simulink library "INT_StSys_Strt"  (R2016b)
settings: Solver=VariableStepAuto  StartTime=0.0  StopTime=10.0  RelTol=1e-3
settings Model: Creator=Administrator  LastModifiedBy=Administrator

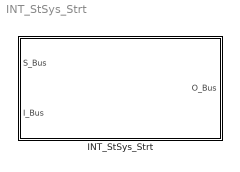
== system INT_StSys_Strt ==
  INT_StSys_Strt : Subsystem

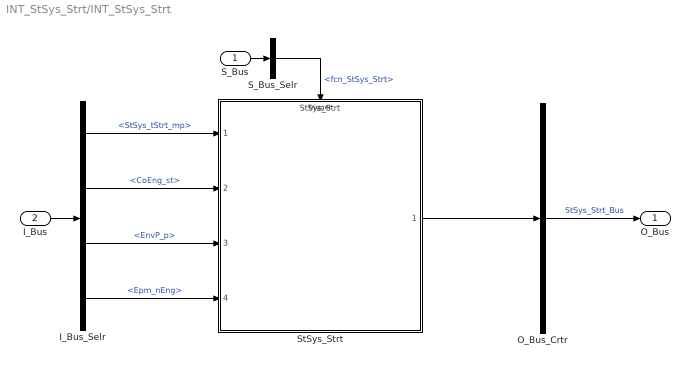
== system INT_StSys_Strt/INT_StSys_Strt ==
  S_Bus : Inport
  I_Bus : Inport  Port=2
  I_Bus_Selr : BusSelector  OutputSignals=StSys_tStrt_mp,CoEng_st,EnvP_p,Epm_nEng
  O_Bus_Crtr : BusCreator  Inputs=1
  S_Bus_Selr : BusSelector  OutputSignals=fcn_StSys_Strt
  StSys_Strt : ModelReference  ModelNameDialog=StSys_Strt  SimulationMode=Normal  ModelReferenceVersion=1.20  TriggerPortName=function  TriggerPortTriggerType=function-call  TriggerPortStatesWhenEnabling=held
  O_Bus : Outport
  wires:
  S_Bus_Selr/1 -> StSys_Strt/Trigger  "<fcn_StSys_Strt>"
  S_Bus/1 -> S_Bus_Selr/1
  I_Bus/1 -> I_Bus_Selr/1
  I_Bus_Selr/1 -> StSys_Strt/1  "<StSys_tStrt_mp>"
  I_Bus_Selr/2 -> StSys_Strt/2  "<CoEng_st>"
  I_Bus_Selr/3 -> StSys_Strt/3  "<EnvP_p>"
  I_Bus_Selr/4 -> StSys_Strt/4  "<Epm_nEng>"
  O_Bus_Crtr/1 -> O_Bus/1  "StSys_Strt_Bus"
  StSys_Strt/1 -> O_Bus_Crtr/1
